simulink model "ACC_Scenario_006_cs"  (R2014b)
settings: Solver=ode5  SolverMode=SingleTasking  StartTime=0.0  StopTime=inf  FixedStep=1/100  RelTol=1e-3
PreLoadFcn:
  | mbxruntime.callbacks.PreLoadFcn(bdroot);
  | check_NUTS_defined;
  | 
  | assignin('base',['model_closed_' bdroot],false);addpath('../includes_ACC');
PostLoadFcn:
  | mbxruntime.callbacks.PostLoadFcn(bdroot);
InitFcn:
  | mbxruntime.callbacks.InitFcn(bdroot);
StartFcn:
  | mbxruntime.callbacks.StartFcn(bdroot);
StopFcn:
  | mbxruntime.callbacks.StopFcn(bdroot);
model workspace: external: MAT-File .\ACC_Scenario_006_cs_hws.mat (data not in the file)
undefined symbols (not defined in the file or in its folder): mbxruntime, OrientationPitch, OrientationRoll, PositionX, PositionY, PositionZ, tabledata, warningInitialVelocity, x0
undefined symbols (not defined in the file): ACC_Scenario_006_cs_061450488d6753c4, ACC_Scenario_006_cs_13896134c615b72a, ACC_Scenario_006_cs_18eaf2a52f2ef75d, ACC_Scenario_006_cs_59e375456829d2f0, ACC_Scenario_006_cs_8a2109b915871f11, ACC_Scenario_006_cs_a4f79cab717c06e2, ACC_Scenario_006_cs_Audi_A8_1_Dynamics_Simple_initialPitch, ACC_Scenario_006_cs_Audi_A8_1_Dynamics_Simple_initialRoll, ACC_Scenario_006_cs_Audi_A8_1_Dynamics_Simple_initialX, ACC_Scenario_006_cs_Audi_A8_1_Dynamics_Simple_initialY, ACC_Scenario_006_cs_Audi_A8_1_Dynamics_Simple_initialYaw, ACC_Scenario_006_cs_Audi_A8_1_Dynamics_Simple_initialZ, ACC_Scenario_006_cs_BMW_X5_1_Path_pathUniqueID, ACC_Scenario_006_cs_BMW_X5_1_SpeedProfile_speedProfileUniqueID, ACC_Scenario_006_cs_e4633c18fd34a832, ACC_Scenario_006_cs_f83c81dc10cd364a, ACC_Scenario_006_cs_Fiat_Bravo_1_Path_pathUniqueID, ACC_Scenario_006_cs_Ford_Fiesta_1_Path_pathUniqueID, ACC_Scenario_006_cs_Honda_Pan_European_1_Path_pathUniqueID, ACC_Scenario_006_cs_Mazda_RX8_1_Path_pathUniqueID, ACC_Scenario_006_cs_Sphere_1_Dynamics_Empty_STATE_Sphere_1_x0, ACC_Scenario_006_cs_Sphere_1_Dynamics_Empty_STATE_Sphere_1_y0, ACC_Scenario_006_cs_Sphere_1_Dynamics_Empty_STATE_Sphere_1_Yaw0, ACC_Scenario_006_cs_Sphere_1_Dynamics_Empty_STATE_Sphere_1_z0, ACC_Scenario_006_cs_Toyota_Yaris_1_Path_pathUniqueID, SteeringColumn, SteeringWheel, Wheel0, Wheel0_Suspension, Wheel1, Wheel1_Suspension, WheelL0, WheelL1, WheelR0, WheelR1
libraries: simulink_extras x60, simulink x21, PreScanSimulinkLibrary x5, PreScanUsefulBlocks x2
(part 16 of 24)

== system ACC_Scenario_006_cs/VISUMatrixSign_HighwayOverhang_1/Actuator ==
  VISUMatrixSign_HighwayOverhang_1 : Inport  Tag=inport/VisuMatrixSign  SampleTime=1/100  BusOutputAsStruct=on
  DemuxVisuMatrixSign : Demux  Outputs=2
  visu_MatrixSign_1 : S-Function  FunctionName=sfun_ResourceNameSelector  Parameters=mbxruntime.parameters.convert(UniqueID), mbxruntime.parameters.convert(ResourceList), mbxruntime.parameters.convert(PivotName),tabledata, TimeStep  EnableBusSupport=off  mask(PreScan Sink Block: VisuMatrixSign){UniqueID=109, ResourceList={'1' 'InformationSign\MatrixSign_GreenArrow.png' '2' 'InformationSign\sign1.jpg' '3' 'InformationSign\sign2.jpg' '4' 'InformationSign\sign3.jpg' '5' 'InformationSign\sign10.png' '7' 'InformationSign\SEARCH_Logo.png' '8' 'InformationSign\sharp_edges.jpg' '9' 'InformationSign\road_surprises.jpg' '10' 'InformationSign\sign5.JPG' '11' 'InformationSign\tacos.jpg' '12' 'InformationSign\dont_even_think.jpg' '13' 'InformationSign\cthulhuwarn.jpg' '14' 'InformationSign\sign7.JPG' '15' 'InformationSign\sign32.jpg' '16' 'InformationSign\NoParking.jpg' '17' 'InformationSign\TheFuture.jpg' '18' 'InformationSign\sign4.jpg' '19' 'InformationSign\sign31.jpg' '20' 'InformationSign\Empty.jpeg' }, PivotName=/child:name=MatrixSign_1/trafficSignElement, TimeStep=1/100}
      mask prompts: UniqueID "Parent Unique Identifier (auto-generated)"; ResourceList "Resource List (auto-generated)"; PivotName "Name of pivot (auto-generated)"; TimeStep "Simulink time step"
      mask help:
      | The VisuMatrixSign block provides a way to adapt the texture of the plates connected to an overhang, based on Resource IDs of the texture files.
      |
      | For more information, please click Help.
      mask init:
      | [tabledata] = mbxruntime.parameters.table(UniqueID,ResourceList,PivotName);
      mask Help: eval('openHelp(733)')
      mask Display: image(imread('HighwaySpeedMatrix.png'))
  visu_MatrixSign_2 : S-Function  FunctionName=sfun_ResourceNameSelector  Parameters=mbxruntime.parameters.convert(UniqueID), mbxruntime.parameters.convert(ResourceList), mbxruntime.parameters.convert(PivotName),tabledata, TimeStep  EnableBusSupport=off  mask(PreScan Sink Block: VisuMatrixSign){UniqueID=109, ResourceList={'1' 'InformationSign\MatrixSign_GreenArrow.png' '2' 'InformationSign\sign1.jpg' '3' 'InformationSign\sign2.jpg' '4' 'InformationSign\sign3.jpg' '5' 'InformationSign\sign10.png' '7' 'InformationSign\SEARCH_Logo.png' '8' 'InformationSign\sharp_edges.jpg' '9' 'InformationSign\road_surprises.jpg' '10' 'InformationSign\sign5.JPG' '11' 'InformationSign\tacos.jpg' '12' 'InformationSign\dont_even_think.jpg' '13' 'InformationSign\cthulhuwarn.jpg' '14' 'InformationSign\sign7.JPG' '15' 'InformationSign\sign32.jpg' '16' 'InformationSign\NoParking.jpg' '17' 'InformationSign\TheFuture.jpg' '18' 'InformationSign\sign4.jpg' '19' 'InformationSign\sign31.jpg' '20' 'InformationSign\Empty.jpeg' }, PivotName=/child:name=MatrixSign_2/trafficSignElement, TimeStep=1/100}
      mask prompts: UniqueID "Parent Unique Identifier (auto-generated)"; ResourceList "Resource List (auto-generated)"; PivotName "Name of pivot (auto-generated)"; TimeStep "Simulink time step"
      mask help:
      | The VisuMatrixSign block provides a way to adapt the texture of the plates connected to an overhang, based on Resource IDs of the texture files.
      |
      | For more information, please click Help.
      mask init:
      | [tabledata] = mbxruntime.parameters.table(UniqueID,ResourceList,PivotName);
      mask Help: eval('openHelp(733)')
      mask Display: image(imread('HighwaySpeedMatrix.png'))
  wires:
  VISUMatrixSign_HighwayOverhang_1/1 -> DemuxVisuMatrixSign/1
  DemuxVisuMatrixSign/1 -> visu_MatrixSign_1/1
  DemuxVisuMatrixSign/2 -> visu_MatrixSign_2/1

== system ACC_Scenario_006_cs/VISUMatrixSign_HighwayOverhang_10/Actuator ==
  VISUMatrixSign_HighwayOverhang_10 : Inport  Tag=inport/VisuMatrixSign  SampleTime=1/100  BusOutputAsStruct=on
  DemuxVisuMatrixSign : Demux  Outputs=2
  visu_InformationPlate_15 : S-Function  FunctionName=sfun_ResourceNameSelector  Parameters=mbxruntime.parameters.convert(UniqueID), mbxruntime.parameters.convert(ResourceList), mbxruntime.parameters.convert(PivotName),tabledata, TimeStep  EnableBusSupport=off  mask(PreScan Sink Block: VisuMatrixSign){UniqueID=119, ResourceList={'1' 'InformationSign\MatrixSign_GreenArrow.png' '2' 'InformationSign\sign1.jpg' '3' 'InformationSign\sign2.jpg' '4' 'InformationSign\sign3.jpg' '5' 'InformationSign\sign10.png' '7' 'InformationSign\SEARCH_Logo.png' '8' 'InformationSign\sharp_edges.jpg' '9' 'InformationSign\road_surprises.jpg' '10' 'InformationSign\sign5.JPG' '11' 'InformationSign\tacos.jpg' '12' 'InformationSign\dont_even_think.jpg' '13' 'InformationSign\cthulhuwarn.jpg' '14' 'InformationSign\sign7.JPG' '15' 'InformationSign\sign32.jpg' '16' 'InformationSign\NoParking.jpg' '17' 'InformationSign\TheFuture.jpg' '18' 'InformationSign\sign4.jpg' '19' 'InformationSign\sign31.jpg' '20' 'InformationSign\Empty.jpeg' }, PivotName=/child:name=HighwayOverhang_10.InformationPlate_15/trafficSignElement, TimeStep=1/100}
      mask prompts: UniqueID "Parent Unique Identifier (auto-generated)"; ResourceList "Resource List (auto-generated)"; PivotName "Name of pivot (auto-generated)"; TimeStep "Simulink time step"
      mask help:
      | The VisuMatrixSign block provides a way to adapt the texture of the plates connected to an overhang, based on Resource IDs of the texture files.
      |
      | For more information, please click Help.
      mask init:
      | [tabledata] = mbxruntime.parameters.table(UniqueID,ResourceList,PivotName);
      mask Help: eval('openHelp(733)')
      mask Display: image(imread('HighwaySpeedMatrix.png'))
  visu_InformationPlate_16 : S-Function  FunctionName=sfun_ResourceNameSelector  Parameters=mbxruntime.parameters.convert(UniqueID), mbxruntime.parameters.convert(ResourceList), mbxruntime.parameters.convert(PivotName),tabledata, TimeStep  EnableBusSupport=off  mask(PreScan Sink Block: VisuMatrixSign){UniqueID=119, ResourceList={'1' 'InformationSign\MatrixSign_GreenArrow.png' '2' 'InformationSign\sign1.jpg' '3' 'InformationSign\sign2.jpg' '4' 'InformationSign\sign3.jpg' '5' 'InformationSign\sign10.png' '7' 'InformationSign\SEARCH_Logo.png' '8' 'InformationSign\sharp_edges.jpg' '9' 'InformationSign\road_surprises.jpg' '10' 'InformationSign\sign5.JPG' '11' 'InformationSign\tacos.jpg' '12' 'InformationSign\dont_even_think.jpg' '13' 'InformationSign\cthulhuwarn.jpg' '14' 'InformationSign\sign7.JPG' '15' 'InformationSign\sign32.jpg' '16' 'InformationSign\NoParking.jpg' '17' 'InformationSign\TheFuture.jpg' '18' 'InformationSign\sign4.jpg' '19' 'InformationSign\sign31.jpg' '20' 'InformationSign\Empty.jpeg' }, PivotName=/child:name=HighwayOverhang_10.InformationPlate_16/trafficSignElement, TimeStep=1/100}
      mask prompts: UniqueID "Parent Unique Identifier (auto-generated)"; ResourceList "Resource List (auto-generated)"; PivotName "Name of pivot (auto-generated)"; TimeStep "Simulink time step"
      mask help:
      | The VisuMatrixSign block provides a way to adapt the texture of the plates connected to an overhang, based on Resource IDs of the texture files.
      |
      | For more information, please click Help.
      mask init:
      | [tabledata] = mbxruntime.parameters.table(UniqueID,ResourceList,PivotName);
      mask Help: eval('openHelp(733)')
      mask Display: image(imread('HighwaySpeedMatrix.png'))
  wires:
  VISUMatrixSign_HighwayOverhang_10/1 -> DemuxVisuMatrixSign/1
  DemuxVisuMatrixSign/1 -> visu_InformationPlate_15/1
  DemuxVisuMatrixSign/2 -> visu_InformationPlate_16/1

== system ACC_Scenario_006_cs/VISUMatrixSign_HighwayOverhang_11/Actuator ==
  VISUMatrixSign_HighwayOverhang_11 : Inport  Tag=inport/VisuMatrixSign  SampleTime=1/100  BusOutputAsStruct=on
  DemuxVisuMatrixSign : Demux  Outputs=2
  visu_MatrixSign_7 : S-Function  FunctionName=sfun_ResourceNameSelector  Parameters=mbxruntime.parameters.convert(UniqueID), mbxruntime.parameters.convert(ResourceList), mbxruntime.parameters.convert(PivotName),tabledata, TimeStep  EnableBusSupport=off  mask(PreScan Sink Block: VisuMatrixSign){UniqueID=120, ResourceList={'1' 'InformationSign\MatrixSign_GreenArrow.png' '2' 'InformationSign\sign1.jpg' '3' 'InformationSign\sign2.jpg' '4' 'InformationSign\sign3.jpg' '5' 'InformationSign\sign10.png' '7' 'InformationSign\SEARCH_Logo.png' '8' 'InformationSign\sharp_edges.jpg' '9' 'InformationSign\road_surprises.jpg' '10' 'InformationSign\sign5.JPG' '11' 'InformationSign\tacos.jpg' '12' 'InformationSign\dont_even_think.jpg' '13' 'InformationSign\cthulhuwarn.jpg' '14' 'InformationSign\sign7.JPG' '15' 'InformationSign\sign32.jpg' '16' 'InformationSign\NoParking.jpg' '17' 'InformationSign\TheFuture.jpg' '18' 'InformationSign\sign4.jpg' '19' 'InformationSign\sign31.jpg' '20' 'InformationSign\Empty.jpeg' }, PivotName=/child:name=MatrixSign_7/trafficSignElement, TimeStep=1/100}
      mask prompts: UniqueID "Parent Unique Identifier (auto-generated)"; ResourceList "Resource List (auto-generated)"; PivotName "Name of pivot (auto-generated)"; TimeStep "Simulink time step"
      mask help:
      | The VisuMatrixSign block provides a way to adapt the texture of the plates connected to an overhang, based on Resource IDs of the texture files.
      |
      | For more information, please click Help.
      mask init:
      | [tabledata] = mbxruntime.parameters.table(UniqueID,ResourceList,PivotName);
      mask Help: eval('openHelp(733)')
      mask Display: image(imread('HighwaySpeedMatrix.png'))
  visu_MatrixSign_8 : S-Function  FunctionName=sfun_ResourceNameSelector  Parameters=mbxruntime.parameters.convert(UniqueID), mbxruntime.parameters.convert(ResourceList), mbxruntime.parameters.convert(PivotName),tabledata, TimeStep  EnableBusSupport=off  mask(PreScan Sink Block: VisuMatrixSign){UniqueID=120, ResourceList={'1' 'InformationSign\MatrixSign_GreenArrow.png' '2' 'InformationSign\sign1.jpg' '3' 'InformationSign\sign2.jpg' '4' 'InformationSign\sign3.jpg' '5' 'InformationSign\sign10.png' '7' 'InformationSign\SEARCH_Logo.png' '8' 'InformationSign\sharp_edges.jpg' '9' 'InformationSign\road_surprises.jpg' '10' 'InformationSign\sign5.JPG' '11' 'InformationSign\tacos.jpg' '12' 'InformationSign\dont_even_think.jpg' '13' 'InformationSign\cthulhuwarn.jpg' '14' 'InformationSign\sign7.JPG' '15' 'InformationSign\sign32.jpg' '16' 'InformationSign\NoParking.jpg' '17' 'InformationSign\TheFuture.jpg' '18' 'InformationSign\sign4.jpg' '19' 'InformationSign\sign31.jpg' '20' 'InformationSign\Empty.jpeg' }, PivotName=/child:name=MatrixSign_8/trafficSignElement, TimeStep=1/100}
      mask prompts: UniqueID "Parent Unique Identifier (auto-generated)"; ResourceList "Resource List (auto-generated)"; PivotName "Name of pivot (auto-generated)"; TimeStep "Simulink time step"
      mask help:
      | The VisuMatrixSign block provides a way to adapt the texture of the plates connected to an overhang, based on Resource IDs of the texture files.
      |
      | For more information, please click Help.
      mask init:
      | [tabledata] = mbxruntime.parameters.table(UniqueID,ResourceList,PivotName);
      mask Help: eval('openHelp(733)')
      mask Display: image(imread('HighwaySpeedMatrix.png'))
  wires:
  VISUMatrixSign_HighwayOverhang_11/1 -> DemuxVisuMatrixSign/1
  DemuxVisuMatrixSign/1 -> visu_MatrixSign_7/1
  DemuxVisuMatrixSign/2 -> visu_MatrixSign_8/1

== system ACC_Scenario_006_cs/VISUMatrixSign_HighwayOverhang_12/Actuator ==
  VISUMatrixSign_HighwayOverhang_12 : Inport  Tag=inport/VisuMatrixSign  SampleTime=1/100  BusOutputAsStruct=on
  DemuxVisuMatrixSign : Demux  Outputs=2
  visu_MatrixSign_5 : S-Function  FunctionName=sfun_ResourceNameSelector  Parameters=mbxruntime.parameters.convert(UniqueID), mbxruntime.parameters.convert(ResourceList), mbxruntime.parameters.convert(PivotName),tabledata, TimeStep  EnableBusSupport=off  mask(PreScan Sink Block: VisuMatrixSign){UniqueID=121, ResourceList={'1' 'InformationSign\MatrixSign_GreenArrow.png' '2' 'InformationSign\sign1.jpg' '3' 'InformationSign\sign2.jpg' '4' 'InformationSign\sign3.jpg' '5' 'InformationSign\sign10.png' '7' 'InformationSign\SEARCH_Logo.png' '8' 'InformationSign\sharp_edges.jpg' '9' 'InformationSign\road_surprises.jpg' '10' 'InformationSign\sign5.JPG' '11' 'InformationSign\tacos.jpg' '12' 'InformationSign\dont_even_think.jpg' '13' 'InformationSign\cthulhuwarn.jpg' '14' 'InformationSign\sign7.JPG' '15' 'InformationSign\sign32.jpg' '16' 'InformationSign\NoParking.jpg' '17' 'InformationSign\TheFuture.jpg' '18' 'InformationSign\sign4.jpg' '19' 'InformationSign\sign31.jpg' '20' 'InformationSign\Empty.jpeg' }, PivotName=/child:name=MatrixSign_5/trafficSignElement, TimeStep=1/100}
      mask prompts: UniqueID "Parent Unique Identifier (auto-generated)"; ResourceList "Resource List (auto-generated)"; PivotName "Name of pivot (auto-generated)"; TimeStep "Simulink time step"
      mask help:
      | The VisuMatrixSign block provides a way to adapt the texture of the plates connected to an overhang, based on Resource IDs of the texture files.
      |
      | For more information, please click Help.
      mask init:
      | [tabledata] = mbxruntime.parameters.table(UniqueID,ResourceList,PivotName);
      mask Help: eval('openHelp(733)')
      mask Display: image(imread('HighwaySpeedMatrix.png'))
  visu_MatrixSign_6 : S-Function  FunctionName=sfun_ResourceNameSelector  Parameters=mbxruntime.parameters.convert(UniqueID), mbxruntime.parameters.convert(ResourceList), mbxruntime.parameters.convert(PivotName),tabledata, TimeStep  EnableBusSupport=off  mask(PreScan Sink Block: VisuMatrixSign){UniqueID=121, ResourceList={'1' 'InformationSign\MatrixSign_GreenArrow.png' '2' 'InformationSign\sign1.jpg' '3' 'InformationSign\sign2.jpg' '4' 'InformationSign\sign3.jpg' '5' 'InformationSign\sign10.png' '7' 'InformationSign\SEARCH_Logo.png' '8' 'InformationSign\sharp_edges.jpg' '9' 'InformationSign\road_surprises.jpg' '10' 'InformationSign\sign5.JPG' '11' 'InformationSign\tacos.jpg' '12' 'InformationSign\dont_even_think.jpg' '13' 'InformationSign\cthulhuwarn.jpg' '14' 'InformationSign\sign7.JPG' '15' 'InformationSign\sign32.jpg' '16' 'InformationSign\NoParking.jpg' '17' 'InformationSign\TheFuture.jpg' '18' 'InformationSign\sign4.jpg' '19' 'InformationSign\sign31.jpg' '20' 'InformationSign\Empty.jpeg' }, PivotName=/child:name=MatrixSign_6/trafficSignElement, TimeStep=1/100}
      mask prompts: UniqueID "Parent Unique Identifier (auto-generated)"; ResourceList "Resource List (auto-generated)"; PivotName "Name of pivot (auto-generated)"; TimeStep "Simulink time step"
      mask help:
      | The VisuMatrixSign block provides a way to adapt the texture of the plates connected to an overhang, based on Resource IDs of the texture files.
      |
      | For more information, please click Help.
      mask init:
      | [tabledata] = mbxruntime.parameters.table(UniqueID,ResourceList,PivotName);
      mask Help: eval('openHelp(733)')
      mask Display: image(imread('HighwaySpeedMatrix.png'))
  wires:
  VISUMatrixSign_HighwayOverhang_12/1 -> DemuxVisuMatrixSign/1
  DemuxVisuMatrixSign/1 -> visu_MatrixSign_5/1
  DemuxVisuMatrixSign/2 -> visu_MatrixSign_6/1

== system ACC_Scenario_006_cs/VISUMatrixSign_HighwayOverhang_2/Actuator ==
  VISUMatrixSign_HighwayOverhang_2 : Inport  Tag=inport/VisuMatrixSign  SampleTime=1/100  BusOutputAsStruct=on
  DemuxVisuMatrixSign : Demux  Outputs=2
  visu_MatrixSign_3 : S-Function  FunctionName=sfun_ResourceNameSelector  Parameters=mbxruntime.parameters.convert(UniqueID), mbxruntime.parameters.convert(ResourceList), mbxruntime.parameters.convert(PivotName),tabledata, TimeStep  EnableBusSupport=off  mask(PreScan Sink Block: VisuMatrixSign){UniqueID=110, ResourceList={'1' 'InformationSign\MatrixSign_GreenArrow.png' '2' 'InformationSign\sign1.jpg' '3' 'InformationSign\sign2.jpg' '4' 'InformationSign\sign3.jpg' '5' 'InformationSign\sign10.png' '7' 'InformationSign\SEARCH_Logo.png' '8' 'InformationSign\sharp_edges.jpg' '9' 'InformationSign\road_surprises.jpg' '10' 'InformationSign\sign5.JPG' '11' 'InformationSign\tacos.jpg' '12' 'InformationSign\dont_even_think.jpg' '13' 'InformationSign\cthulhuwarn.jpg' '14' 'InformationSign\sign7.JPG' '15' 'InformationSign\sign32.jpg' '16' 'InformationSign\NoParking.jpg' '17' 'InformationSign\TheFuture.jpg' '18' 'InformationSign\sign4.jpg' '19' 'InformationSign\sign31.jpg' '20' 'InformationSign\Empty.jpeg' }, PivotName=/child:name=MatrixSign_3/trafficSignElement, TimeStep=1/100}
      mask prompts: UniqueID "Parent Unique Identifier (auto-generated)"; ResourceList "Resource List (auto-generated)"; PivotName "Name of pivot (auto-generated)"; TimeStep "Simulink time step"
      mask help:
      | The VisuMatrixSign block provides a way to adapt the texture of the plates connected to an overhang, based on Resource IDs of the texture files.
      |
      | For more information, please click Help.
      mask init:
      | [tabledata] = mbxruntime.parameters.table(UniqueID,ResourceList,PivotName);
      mask Help: eval('openHelp(733)')
      mask Display: image(imread('HighwaySpeedMatrix.png'))
  visu_MatrixSign_4 : S-Function  FunctionName=sfun_ResourceNameSelector  Parameters=mbxruntime.parameters.convert(UniqueID), mbxruntime.parameters.convert(ResourceList), mbxruntime.parameters.convert(PivotName),tabledata, TimeStep  EnableBusSupport=off  mask(PreScan Sink Block: VisuMatrixSign){UniqueID=110, ResourceList={'1' 'InformationSign\MatrixSign_GreenArrow.png' '2' 'InformationSign\sign1.jpg' '3' 'InformationSign\sign2.jpg' '4' 'InformationSign\sign3.jpg' '5' 'InformationSign\sign10.png' '7' 'InformationSign\SEARCH_Logo.png' '8' 'InformationSign\sharp_edges.jpg' '9' 'InformationSign\road_surprises.jpg' '10' 'InformationSign\sign5.JPG' '11' 'InformationSign\tacos.jpg' '12' 'InformationSign\dont_even_think.jpg' '13' 'InformationSign\cthulhuwarn.jpg' '14' 'InformationSign\sign7.JPG' '15' 'InformationSign\sign32.jpg' '16' 'InformationSign\NoParking.jpg' '17' 'InformationSign\TheFuture.jpg' '18' 'InformationSign\sign4.jpg' '19' 'InformationSign\sign31.jpg' '20' 'InformationSign\Empty.jpeg' }, PivotName=/child:name=MatrixSign_4/trafficSignElement, TimeStep=1/100}
      mask prompts: UniqueID "Parent Unique Identifier (auto-generated)"; ResourceList "Resource List (auto-generated)"; PivotName "Name of pivot (auto-generated)"; TimeStep "Simulink time step"
      mask help:
      | The VisuMatrixSign block provides a way to adapt the texture of the plates connected to an overhang, based on Resource IDs of the texture files.
      |
      | For more information, please click Help.
      mask init:
      | [tabledata] = mbxruntime.parameters.table(UniqueID,ResourceList,PivotName);
      mask Help: eval('openHelp(733)')
      mask Display: image(imread('HighwaySpeedMatrix.png'))
  wires:
  VISUMatrixSign_HighwayOverhang_2/1 -> DemuxVisuMatrixSign/1
  DemuxVisuMatrixSign/1 -> visu_MatrixSign_3/1
  DemuxVisuMatrixSign/2 -> visu_MatrixSign_4/1

== system ACC_Scenario_006_cs/VISUMatrixSign_HighwayOverhang_3/Actuator ==
  VISUMatrixSign_HighwayOverhang_3 : Inport  Tag=inport/VisuMatrixSign  SampleTime=1/100  BusOutputAsStruct=on
  DemuxVisuMatrixSign : Demux  Outputs=2
  visu_InformationPlate_1 : S-Function  FunctionName=sfun_ResourceNameSelector  Parameters=mbxruntime.parameters.convert(UniqueID), mbxruntime.parameters.convert(ResourceList), mbxruntime.parameters.convert(PivotName),tabledata, TimeStep  EnableBusSupport=off  mask(PreScan Sink Block: VisuMatrixSign){UniqueID=112, ResourceList={'1' 'InformationSign\MatrixSign_GreenArrow.png' '2' 'InformationSign\sign1.jpg' '3' 'InformationSign\sign2.jpg' '4' 'InformationSign\sign3.jpg' '5' 'InformationSign\sign10.png' '7' 'InformationSign\SEARCH_Logo.png' '8' 'InformationSign\sharp_edges.jpg' '9' 'InformationSign\road_surprises.jpg' '10' 'InformationSign\sign5.JPG' '11' 'InformationSign\tacos.jpg' '12' 'InformationSign\dont_even_think.jpg' '13' 'InformationSign\cthulhuwarn.jpg' '14' 'InformationSign\sign7.JPG' '15' 'InformationSign\sign32.jpg' '16' 'InformationSign\NoParking.jpg' '17' 'InformationSign\TheFuture.jpg' '18' 'InformationSign\sign4.jpg' '19' 'InformationSign\sign31.jpg' '20' 'InformationSign\Empty.jpeg' }, PivotName=/child:name=HighwayOverhang_3.InformationPlate_1/trafficSignElement, TimeStep=1/100}
      mask prompts: UniqueID "Parent Unique Identifier (auto-generated)"; ResourceList "Resource List (auto-generated)"; PivotName "Name of pivot (auto-generated)"; TimeStep "Simulink time step"
      mask help:
      | The VisuMatrixSign block provides a way to adapt the texture of the plates connected to an overhang, based on Resource IDs of the texture files.
      |
      | For more information, please click Help.
      mask init:
      | [tabledata] = mbxruntime.parameters.table(UniqueID,ResourceList,PivotName);
      mask Help: eval('openHelp(733)')
      mask Display: image(imread('HighwaySpeedMatrix.png'))
  visu_InformationPlate_2 : S-Function  FunctionName=sfun_ResourceNameSelector  Parameters=mbxruntime.parameters.convert(UniqueID), mbxruntime.parameters.convert(ResourceList), mbxruntime.parameters.convert(PivotName),tabledata, TimeStep  EnableBusSupport=off  mask(PreScan Sink Block: VisuMatrixSign){UniqueID=112, ResourceList={'1' 'InformationSign\MatrixSign_GreenArrow.png' '2' 'InformationSign\sign1.jpg' '3' 'InformationSign\sign2.jpg' '4' 'InformationSign\sign3.jpg' '5' 'InformationSign\sign10.png' '7' 'InformationSign\SEARCH_Logo.png' '8' 'InformationSign\sharp_edges.jpg' '9' 'InformationSign\road_surprises.jpg' '10' 'InformationSign\sign5.JPG' '11' 'InformationSign\tacos.jpg' '12' 'InformationSign\dont_even_think.jpg' '13' 'InformationSign\cthulhuwarn.jpg' '14' 'InformationSign\sign7.JPG' '15' 'InformationSign\sign32.jpg' '16' 'InformationSign\NoParking.jpg' '17' 'InformationSign\TheFuture.jpg' '18' 'InformationSign\sign4.jpg' '19' 'InformationSign\sign31.jpg' '20' 'InformationSign\Empty.jpeg' }, PivotName=/child:name=HighwayOverhang_3.InformationPlate_2/trafficSignElement, TimeStep=1/100}
      mask prompts: UniqueID "Parent Unique Identifier (auto-generated)"; ResourceList "Resource List (auto-generated)"; PivotName "Name of pivot (auto-generated)"; TimeStep "Simulink time step"
      mask help:
      | The VisuMatrixSign block provides a way to adapt the texture of the plates connected to an overhang, based on Resource IDs of the texture files.
      |
      | For more information, please click Help.
      mask init:
      | [tabledata] = mbxruntime.parameters.table(UniqueID,ResourceList,PivotName);
      mask Help: eval('openHelp(733)')
      mask Display: image(imread('HighwaySpeedMatrix.png'))
  wires:
  VISUMatrixSign_HighwayOverhang_3/1 -> DemuxVisuMatrixSign/1
  DemuxVisuMatrixSign/1 -> visu_InformationPlate_1/1
  DemuxVisuMatrixSign/2 -> visu_InformationPlate_2/1

== system ACC_Scenario_006_cs/VISUMatrixSign_HighwayOverhang_4/Actuator ==
  VISUMatrixSign_HighwayOverhang_4 : Inport  Tag=inport/VisuMatrixSign  SampleTime=1/100  BusOutputAsStruct=on
  DemuxVisuMatrixSign : Demux  Outputs=2
  visu_InformationPlate_3 : S-Function  FunctionName=sfun_ResourceNameSelector  Parameters=mbxruntime.parameters.convert(UniqueID), mbxruntime.parameters.convert(ResourceList), mbxruntime.parameters.convert(PivotName),tabledata, TimeStep  EnableBusSupport=off  mask(PreScan Sink Block: VisuMatrixSign){UniqueID=113, ResourceList={'1' 'InformationSign\MatrixSign_GreenArrow.png' '2' 'InformationSign\sign1.jpg' '3' 'InformationSign\sign2.jpg' '4' 'InformationSign\sign3.jpg' '5' 'InformationSign\sign10.png' '7' 'InformationSign\SEARCH_Logo.png' '8' 'InformationSign\sharp_edges.jpg' '9' 'InformationSign\road_surprises.jpg' '10' 'InformationSign\sign5.JPG' '11' 'InformationSign\tacos.jpg' '12' 'InformationSign\dont_even_think.jpg' '13' 'InformationSign\cthulhuwarn.jpg' '14' 'InformationSign\sign7.JPG' '15' 'InformationSign\sign32.jpg' '16' 'InformationSign\NoParking.jpg' '17' 'InformationSign\TheFuture.jpg' '18' 'InformationSign\sign4.jpg' '19' 'InformationSign\sign31.jpg' '20' 'InformationSign\Empty.jpeg' }, PivotName=/child:name=HighwayOverhang_4.InformationPlate_3/trafficSignElement, TimeStep=1/100}
      mask prompts: UniqueID "Parent Unique Identifier (auto-generated)"; ResourceList "Resource List (auto-generated)"; PivotName "Name of pivot (auto-generated)"; TimeStep "Simulink time step"
      mask help:
      | The VisuMatrixSign block provides a way to adapt the texture of the plates connected to an overhang, based on Resource IDs of the texture files.
      |
      | For more information, please click Help.
      mask init:
      | [tabledata] = mbxruntime.parameters.table(UniqueID,ResourceList,PivotName);
      mask Help: eval('openHelp(733)')
      mask Display: image(imread('HighwaySpeedMatrix.png'))
  visu_InformationPlate_4 : S-Function  FunctionName=sfun_ResourceNameSelector  Parameters=mbxruntime.parameters.convert(UniqueID), mbxruntime.parameters.convert(ResourceList), mbxruntime.parameters.convert(PivotName),tabledata, TimeStep  EnableBusSupport=off  mask(PreScan Sink Block: VisuMatrixSign){UniqueID=113, ResourceList={'1' 'InformationSign\MatrixSign_GreenArrow.png' '2' 'InformationSign\sign1.jpg' '3' 'InformationSign\sign2.jpg' '4' 'InformationSign\sign3.jpg' '5' 'InformationSign\sign10.png' '7' 'InformationSign\SEARCH_Logo.png' '8' 'InformationSign\sharp_edges.jpg' '9' 'InformationSign\road_surprises.jpg' '10' 'InformationSign\sign5.JPG' '11' 'InformationSign\tacos.jpg' '12' 'InformationSign\dont_even_think.jpg' '13' 'InformationSign\cthulhuwarn.jpg' '14' 'InformationSign\sign7.JPG' '15' 'InformationSign\sign32.jpg' '16' 'InformationSign\NoParking.jpg' '17' 'InformationSign\TheFuture.jpg' '18' 'InformationSign\sign4.jpg' '19' 'InformationSign\sign31.jpg' '20' 'InformationSign\Empty.jpeg' }, PivotName=/child:name=HighwayOverhang_4.InformationPlate_4/trafficSignElement, TimeStep=1/100}
      mask prompts: UniqueID "Parent Unique Identifier (auto-generated)"; ResourceList "Resource List (auto-generated)"; PivotName "Name of pivot (auto-generated)"; TimeStep "Simulink time step"
      mask help:
      | The VisuMatrixSign block provides a way to adapt the texture of the plates connected to an overhang, based on Resource IDs of the texture files.
      |
      | For more information, please click Help.
      mask init:
      | [tabledata] = mbxruntime.parameters.table(UniqueID,ResourceList,PivotName);
      mask Help: eval('openHelp(733)')
      mask Display: image(imread('HighwaySpeedMatrix.png'))
  wires:
  VISUMatrixSign_HighwayOverhang_4/1 -> DemuxVisuMatrixSign/1
  DemuxVisuMatrixSign/1 -> visu_InformationPlate_3/1
  DemuxVisuMatrixSign/2 -> visu_InformationPlate_4/1

== system ACC_Scenario_006_cs/VISUMatrixSign_HighwayOverhang_5/Actuator ==
  VISUMatrixSign_HighwayOverhang_5 : Inport  Tag=inport/VisuMatrixSign  SampleTime=1/100  BusOutputAsStruct=on
  DemuxVisuMatrixSign : Demux  Outputs=2
  visu_InformationPlate_5 : S-Function  FunctionName=sfun_ResourceNameSelector  Parameters=mbxruntime.parameters.convert(UniqueID), mbxruntime.parameters.convert(ResourceList), mbxruntime.parameters.convert(PivotName),tabledata, TimeStep  EnableBusSupport=off  mask(PreScan Sink Block: VisuMatrixSign){UniqueID=114, ResourceList={'1' 'InformationSign\MatrixSign_GreenArrow.png' '2' 'InformationSign\sign1.jpg' '3' 'InformationSign\sign2.jpg' '4' 'InformationSign\sign3.jpg' '5' 'InformationSign\sign10.png' '7' 'InformationSign\SEARCH_Logo.png' '8' 'InformationSign\sharp_edges.jpg' '9' 'InformationSign\road_surprises.jpg' '10' 'InformationSign\sign5.JPG' '11' 'InformationSign\tacos.jpg' '12' 'InformationSign\dont_even_think.jpg' '13' 'InformationSign\cthulhuwarn.jpg' '14' 'InformationSign\sign7.JPG' '15' 'InformationSign\sign32.jpg' '16' 'InformationSign\NoParking.jpg' '17' 'InformationSign\TheFuture.jpg' '18' 'InformationSign\sign4.jpg' '19' 'InformationSign\sign31.jpg' '20' 'InformationSign\Empty.jpeg' }, PivotName=/child:name=HighwayOverhang_5.InformationPlate_5/trafficSignElement, TimeStep=1/100}
      mask prompts: UniqueID "Parent Unique Identifier (auto-generated)"; ResourceList "Resource List (auto-generated)"; PivotName "Name of pivot (auto-generated)"; TimeStep "Simulink time step"
      mask help:
      | The VisuMatrixSign block provides a way to adapt the texture of the plates connected to an overhang, based on Resource IDs of the texture files.
      |
      | For more information, please click Help.
      mask init:
      | [tabledata] = mbxruntime.parameters.table(UniqueID,ResourceList,PivotName);
      mask Help: eval('openHelp(733)')
      mask Display: image(imread('HighwaySpeedMatrix.png'))
  visu_InformationPlate_6 : S-Function  FunctionName=sfun_ResourceNameSelector  Parameters=mbxruntime.parameters.convert(UniqueID), mbxruntime.parameters.convert(ResourceList), mbxruntime.parameters.convert(PivotName),tabledata, TimeStep  EnableBusSupport=off  mask(PreScan Sink Block: VisuMatrixSign){UniqueID=114, ResourceList={'1' 'InformationSign\MatrixSign_GreenArrow.png' '2' 'InformationSign\sign1.jpg' '3' 'InformationSign\sign2.jpg' '4' 'InformationSign\sign3.jpg' '5' 'InformationSign\sign10.png' '7' 'InformationSign\SEARCH_Logo.png' '8' 'InformationSign\sharp_edges.jpg' '9' 'InformationSign\road_surprises.jpg' '10' 'InformationSign\sign5.JPG' '11' 'InformationSign\tacos.jpg' '12' 'InformationSign\dont_even_think.jpg' '13' 'InformationSign\cthulhuwarn.jpg' '14' 'InformationSign\sign7.JPG' '15' 'InformationSign\sign32.jpg' '16' 'InformationSign\NoParking.jpg' '17' 'InformationSign\TheFuture.jpg' '18' 'InformationSign\sign4.jpg' '19' 'InformationSign\sign31.jpg' '20' 'InformationSign\Empty.jpeg' }, PivotName=/child:name=HighwayOverhang_5.InformationPlate_6/trafficSignElement, TimeStep=1/100}
      mask prompts: UniqueID "Parent Unique Identifier (auto-generated)"; ResourceList "Resource List (auto-generated)"; PivotName "Name of pivot (auto-generated)"; TimeStep "Simulink time step"
      mask help:
      | The VisuMatrixSign block provides a way to adapt the texture of the plates connected to an overhang, based on Resource IDs of the texture files.
      |
      | For more information, please click Help.
      mask init:
      | [tabledata] = mbxruntime.parameters.table(UniqueID,ResourceList,PivotName);
      mask Help: eval('openHelp(733)')
      mask Display: image(imread('HighwaySpeedMatrix.png'))
  wires:
  VISUMatrixSign_HighwayOverhang_5/1 -> DemuxVisuMatrixSign/1
  DemuxVisuMatrixSign/1 -> visu_InformationPlate_5/1
  DemuxVisuMatrixSign/2 -> visu_InformationPlate_6/1

== system ACC_Scenario_006_cs/VISUMatrixSign_HighwayOverhang_6/Actuator ==
  VISUMatrixSign_HighwayOverhang_6 : Inport  Tag=inport/VisuMatrixSign  SampleTime=1/100  BusOutputAsStruct=on
  DemuxVisuMatrixSign : Demux  Outputs=2
  visu_InformationPlate_7 : S-Function  FunctionName=sfun_ResourceNameSelector  Parameters=mbxruntime.parameters.convert(UniqueID), mbxruntime.parameters.convert(ResourceList), mbxruntime.parameters.convert(PivotName),tabledata, TimeStep  EnableBusSupport=off  mask(PreScan Sink Block: VisuMatrixSign){UniqueID=115, ResourceList={'1' 'InformationSign\MatrixSign_GreenArrow.png' '2' 'InformationSign\sign1.jpg' '3' 'InformationSign\sign2.jpg' '4' 'InformationSign\sign3.jpg' '5' 'InformationSign\sign10.png' '7' 'InformationSign\SEARCH_Logo.png' '8' 'InformationSign\sharp_edges.jpg' '9' 'InformationSign\road_surprises.jpg' '10' 'InformationSign\sign5.JPG' '11' 'InformationSign\tacos.jpg' '12' 'InformationSign\dont_even_think.jpg' '13' 'InformationSign\cthulhuwarn.jpg' '14' 'InformationSign\sign7.JPG' '15' 'InformationSign\sign32.jpg' '16' 'InformationSign\NoParking.jpg' '17' 'InformationSign\TheFuture.jpg' '18' 'InformationSign\sign4.jpg' '19' 'InformationSign\sign31.jpg' '20' 'InformationSign\Empty.jpeg' }, PivotName=/child:name=HighwayOverhang_6.InformationPlate_7/trafficSignElement, TimeStep=1/100}
      mask prompts: UniqueID "Parent Unique Identifier (auto-generated)"; ResourceList "Resource List (auto-generated)"; PivotName "Name of pivot (auto-generated)"; TimeStep "Simulink time step"
      mask help:
      | The VisuMatrixSign block provides a way to adapt the texture of the plates connected to an overhang, based on Resource IDs of the texture files.
      |
      | For more information, please click Help.
      mask init:
      | [tabledata] = mbxruntime.parameters.table(UniqueID,ResourceList,PivotName);
      mask Help: eval('openHelp(733)')
      mask Display: image(imread('HighwaySpeedMatrix.png'))
  visu_InformationPlate_8 : S-Function  FunctionName=sfun_ResourceNameSelector  Parameters=mbxruntime.parameters.convert(UniqueID), mbxruntime.parameters.convert(ResourceList), mbxruntime.parameters.convert(PivotName),tabledata, TimeStep  EnableBusSupport=off  mask(PreScan Sink Block: VisuMatrixSign){UniqueID=115, ResourceList={'1' 'InformationSign\MatrixSign_GreenArrow.png' '2' 'InformationSign\sign1.jpg' '3' 'InformationSign\sign2.jpg' '4' 'InformationSign\sign3.jpg' '5' 'InformationSign\sign10.png' '7' 'InformationSign\SEARCH_Logo.png' '8' 'InformationSign\sharp_edges.jpg' '9' 'InformationSign\road_surprises.jpg' '10' 'InformationSign\sign5.JPG' '11' 'InformationSign\tacos.jpg' '12' 'InformationSign\dont_even_think.jpg' '13' 'InformationSign\cthulhuwarn.jpg' '14' 'InformationSign\sign7.JPG' '15' 'InformationSign\sign32.jpg' '16' 'InformationSign\NoParking.jpg' '17' 'InformationSign\TheFuture.jpg' '18' 'InformationSign\sign4.jpg' '19' 'InformationSign\sign31.jpg' '20' 'InformationSign\Empty.jpeg' }, PivotName=/child:name=HighwayOverhang_6.InformationPlate_8/trafficSignElement, TimeStep=1/100}
      mask prompts: UniqueID "Parent Unique Identifier (auto-generated)"; ResourceList "Resource List (auto-generated)"; PivotName "Name of pivot (auto-generated)"; TimeStep "Simulink time step"
      mask help:
      | The VisuMatrixSign block provides a way to adapt the texture of the plates connected to an overhang, based on Resource IDs of the texture files.
      |
      | For more information, please click Help.
      mask init:
      | [tabledata] = mbxruntime.parameters.table(UniqueID,ResourceList,PivotName);
      mask Help: eval('openHelp(733)')
      mask Display: image(imread('HighwaySpeedMatrix.png'))
  wires:
  VISUMatrixSign_HighwayOverhang_6/1 -> DemuxVisuMatrixSign/1
  DemuxVisuMatrixSign/1 -> visu_InformationPlate_7/1
  DemuxVisuMatrixSign/2 -> visu_InformationPlate_8/1

== system ACC_Scenario_006_cs/VISUMatrixSign_HighwayOverhang_7/Actuator ==
  VISUMatrixSign_HighwayOverhang_7 : Inport  Tag=inport/VisuMatrixSign  SampleTime=1/100  BusOutputAsStruct=on
  DemuxVisuMatrixSign : Demux  Outputs=2
  visu_InformationPlate_10 : S-Function  FunctionName=sfun_ResourceNameSelector  Parameters=mbxruntime.parameters.convert(UniqueID), mbxruntime.parameters.convert(ResourceList), mbxruntime.parameters.convert(PivotName),tabledata, TimeStep  EnableBusSupport=off  mask(PreScan Sink Block: VisuMatrixSign){UniqueID=116, ResourceList={'1' 'InformationSign\MatrixSign_GreenArrow.png' '2' 'InformationSign\sign1.jpg' '3' 'InformationSign\sign2.jpg' '4' 'InformationSign\sign3.jpg' '5' 'InformationSign\sign10.png' '7' 'InformationSign\SEARCH_Logo.png' '8' 'InformationSign\sharp_edges.jpg' '9' 'InformationSign\road_surprises.jpg' '10' 'InformationSign\sign5.JPG' '11' 'InformationSign\tacos.jpg' '12' 'InformationSign\dont_even_think.jpg' '13' 'InformationSign\cthulhuwarn.jpg' '14' 'InformationSign\sign7.JPG' '15' 'InformationSign\sign32.jpg' '16' 'InformationSign\NoParking.jpg' '17' 'InformationSign\TheFuture.jpg' '18' 'InformationSign\sign4.jpg' '19' 'InformationSign\sign31.jpg' '20' 'InformationSign\Empty.jpeg' }, PivotName=/child:name=HighwayOverhang_7.InformationPlate_10/trafficSignElement, TimeStep=1/100}
      mask prompts: UniqueID "Parent Unique Identifier (auto-generated)"; ResourceList "Resource List (auto-generated)"; PivotName "Name of pivot (auto-generated)"; TimeStep "Simulink time step"
      mask help:
      | The VisuMatrixSign block provides a way to adapt the texture of the plates connected to an overhang, based on Resource IDs of the texture files.
      |
      | For more information, please click Help.
      mask init:
      | [tabledata] = mbxruntime.parameters.table(UniqueID,ResourceList,PivotName);
      mask Help: eval('openHelp(733)')
      mask Display: image(imread('HighwaySpeedMatrix.png'))
  visu_InformationPlate_9 : S-Function  FunctionName=sfun_ResourceNameSelector  Parameters=mbxruntime.parameters.convert(UniqueID), mbxruntime.parameters.convert(ResourceList), mbxruntime.parameters.convert(PivotName),tabledata, TimeStep  EnableBusSupport=off  mask(PreScan Sink Block: VisuMatrixSign){UniqueID=116, ResourceList={'1' 'InformationSign\MatrixSign_GreenArrow.png' '2' 'InformationSign\sign1.jpg' '3' 'InformationSign\sign2.jpg' '4' 'InformationSign\sign3.jpg' '5' 'InformationSign\sign10.png' '7' 'InformationSign\SEARCH_Logo.png' '8' 'InformationSign\sharp_edges.jpg' '9' 'InformationSign\road_surprises.jpg' '10' 'InformationSign\sign5.JPG' '11' 'InformationSign\tacos.jpg' '12' 'InformationSign\dont_even_think.jpg' '13' 'InformationSign\cthulhuwarn.jpg' '14' 'InformationSign\sign7.JPG' '15' 'InformationSign\sign32.jpg' '16' 'InformationSign\NoParking.jpg' '17' 'InformationSign\TheFuture.jpg' '18' 'InformationSign\sign4.jpg' '19' 'InformationSign\sign31.jpg' '20' 'InformationSign\Empty.jpeg' }, PivotName=/child:name=HighwayOverhang_7.InformationPlate_9/trafficSignElement, TimeStep=1/100}
      mask prompts: UniqueID "Parent Unique Identifier (auto-generated)"; ResourceList "Resource List (auto-generated)"; PivotName "Name of pivot (auto-generated)"; TimeStep "Simulink time step"
      mask help:
      | The VisuMatrixSign block provides a way to adapt the texture of the plates connected to an overhang, based on Resource IDs of the texture files.
      |
      | For more information, please click Help.
      mask init:
      | [tabledata] = mbxruntime.parameters.table(UniqueID,ResourceList,PivotName);
      mask Help: eval('openHelp(733)')
      mask Display: image(imread('HighwaySpeedMatrix.png'))
  wires:
  VISUMatrixSign_HighwayOverhang_7/1 -> DemuxVisuMatrixSign/1
  DemuxVisuMatrixSign/1 -> visu_InformationPlate_9/1
  DemuxVisuMatrixSign/2 -> visu_InformationPlate_10/1

== system ACC_Scenario_006_cs/VISUMatrixSign_HighwayOverhang_8/Actuator ==
  VISUMatrixSign_HighwayOverhang_8 : Inport  Tag=inport/VisuMatrixSign  SampleTime=1/100  BusOutputAsStruct=on
  DemuxVisuMatrixSign : Demux  Outputs=2
  visu_InformationPlate_11 : S-Function  FunctionName=sfun_ResourceNameSelector  Parameters=mbxruntime.parameters.convert(UniqueID), mbxruntime.parameters.convert(ResourceList), mbxruntime.parameters.convert(PivotName),tabledata, TimeStep  EnableBusSupport=off  mask(PreScan Sink Block: VisuMatrixSign){UniqueID=117, ResourceList={'1' 'InformationSign\MatrixSign_GreenArrow.png' '2' 'InformationSign\sign1.jpg' '3' 'InformationSign\sign2.jpg' '4' 'InformationSign\sign3.jpg' '5' 'InformationSign\sign10.png' '7' 'InformationSign\SEARCH_Logo.png' '8' 'InformationSign\sharp_edges.jpg' '9' 'InformationSign\road_surprises.jpg' '10' 'InformationSign\sign5.JPG' '11' 'InformationSign\tacos.jpg' '12' 'InformationSign\dont_even_think.jpg' '13' 'InformationSign\cthulhuwarn.jpg' '14' 'InformationSign\sign7.JPG' '15' 'InformationSign\sign32.jpg' '16' 'InformationSign\NoParking.jpg' '17' 'InformationSign\TheFuture.jpg' '18' 'InformationSign\sign4.jpg' '19' 'InformationSign\sign31.jpg' '20' 'InformationSign\Empty.jpeg' }, PivotName=/child:name=HighwayOverhang_8.InformationPlate_11/trafficSignElement, TimeStep=1/100}
      mask prompts: UniqueID "Parent Unique Identifier (auto-generated)"; ResourceList "Resource List (auto-generated)"; PivotName "Name of pivot (auto-generated)"; TimeStep "Simulink time step"
      mask help:
      | The VisuMatrixSign block provides a way to adapt the texture of the plates connected to an overhang, based on Resource IDs of the texture files.
      |
      | For more information, please click Help.
      mask init:
      | [tabledata] = mbxruntime.parameters.table(UniqueID,ResourceList,PivotName);
      mask Help: eval('openHelp(733)')
      mask Display: image(imread('HighwaySpeedMatrix.png'))
  visu_InformationPlate_12 : S-Function  FunctionName=sfun_ResourceNameSelector  Parameters=mbxruntime.parameters.convert(UniqueID), mbxruntime.parameters.convert(ResourceList), mbxruntime.parameters.convert(PivotName),tabledata, TimeStep  EnableBusSupport=off  mask(PreScan Sink Block: VisuMatrixSign){UniqueID=117, ResourceList={'1' 'InformationSign\MatrixSign_GreenArrow.png' '2' 'InformationSign\sign1.jpg' '3' 'InformationSign\sign2.jpg' '4' 'InformationSign\sign3.jpg' '5' 'InformationSign\sign10.png' '7' 'InformationSign\SEARCH_Logo.png' '8' 'InformationSign\sharp_edges.jpg' '9' 'InformationSign\road_surprises.jpg' '10' 'InformationSign\sign5.JPG' '11' 'InformationSign\tacos.jpg' '12' 'InformationSign\dont_even_think.jpg' '13' 'InformationSign\cthulhuwarn.jpg' '14' 'InformationSign\sign7.JPG' '15' 'InformationSign\sign32.jpg' '16' 'InformationSign\NoParking.jpg' '17' 'InformationSign\TheFuture.jpg' '18' 'InformationSign\sign4.jpg' '19' 'InformationSign\sign31.jpg' '20' 'InformationSign\Empty.jpeg' }, PivotName=/child:name=HighwayOverhang_8.InformationPlate_12/trafficSignElement, TimeStep=1/100}
      mask prompts: UniqueID "Parent Unique Identifier (auto-generated)"; ResourceList "Resource List (auto-generated)"; PivotName "Name of pivot (auto-generated)"; TimeStep "Simulink time step"
      mask help:
      | The VisuMatrixSign block provides a way to adapt the texture of the plates connected to an overhang, based on Resource IDs of the texture files.
      |
      | For more information, please click Help.
      mask init:
      | [tabledata] = mbxruntime.parameters.table(UniqueID,ResourceList,PivotName);
      mask Help: eval('openHelp(733)')
      mask Display: image(imread('HighwaySpeedMatrix.png'))
  wires:
  VISUMatrixSign_HighwayOverhang_8/1 -> DemuxVisuMatrixSign/1
  DemuxVisuMatrixSign/1 -> visu_InformationPlate_11/1
  DemuxVisuMatrixSign/2 -> visu_InformationPlate_12/1

== system ACC_Scenario_006_cs/VISUMatrixSign_HighwayOverhang_9/Actuator ==
  VISUMatrixSign_HighwayOverhang_9 : Inport  Tag=inport/VisuMatrixSign  SampleTime=1/100  BusOutputAsStruct=on
  DemuxVisuMatrixSign : Demux  Outputs=2
  visu_InformationPlate_13 : S-Function  FunctionName=sfun_ResourceNameSelector  Parameters=mbxruntime.parameters.convert(UniqueID), mbxruntime.parameters.convert(ResourceList), mbxruntime.parameters.convert(PivotName),tabledata, TimeStep  EnableBusSupport=off  mask(PreScan Sink Block: VisuMatrixSign){UniqueID=118, ResourceList={'1' 'InformationSign\MatrixSign_GreenArrow.png' '2' 'InformationSign\sign1.jpg' '3' 'InformationSign\sign2.jpg' '4' 'InformationSign\sign3.jpg' '5' 'InformationSign\sign10.png' '7' 'InformationSign\SEARCH_Logo.png' '8' 'InformationSign\sharp_edges.jpg' '9' 'InformationSign\road_surprises.jpg' '10' 'InformationSign\sign5.JPG' '11' 'InformationSign\tacos.jpg' '12' 'InformationSign\dont_even_think.jpg' '13' 'InformationSign\cthulhuwarn.jpg' '14' 'InformationSign\sign7.JPG' '15' 'InformationSign\sign32.jpg' '16' 'InformationSign\NoParking.jpg' '17' 'InformationSign\TheFuture.jpg' '18' 'InformationSign\sign4.jpg' '19' 'InformationSign\sign31.jpg' '20' 'InformationSign\Empty.jpeg' }, PivotName=/child:name=HighwayOverhang_9.InformationPlate_13/trafficSignElement, TimeStep=1/100}
      mask prompts: UniqueID "Parent Unique Identifier (auto-generated)"; ResourceList "Resource List (auto-generated)"; PivotName "Name of pivot (auto-generated)"; TimeStep "Simulink time step"
      mask help:
      | The VisuMatrixSign block provides a way to adapt the texture of the plates connected to an overhang, based on Resource IDs of the texture files.
      |
      | For more information, please click Help.
      mask init:
      | [tabledata] = mbxruntime.parameters.table(UniqueID,ResourceList,PivotName);
      mask Help: eval('openHelp(733)')
      mask Display: image(imread('HighwaySpeedMatrix.png'))
  visu_InformationPlate_14 : S-Function  FunctionName=sfun_ResourceNameSelector  Parameters=mbxruntime.parameters.convert(UniqueID), mbxruntime.parameters.convert(ResourceList), mbxruntime.parameters.convert(PivotName),tabledata, TimeStep  EnableBusSupport=off  mask(PreScan Sink Block: VisuMatrixSign){UniqueID=118, ResourceList={'1' 'InformationSign\MatrixSign_GreenArrow.png' '2' 'InformationSign\sign1.jpg' '3' 'InformationSign\sign2.jpg' '4' 'InformationSign\sign3.jpg' '5' 'InformationSign\sign10.png' '7' 'InformationSign\SEARCH_Logo.png' '8' 'InformationSign\sharp_edges.jpg' '9' 'InformationSign\road_surprises.jpg' '10' 'InformationSign\sign5.JPG' '11' 'InformationSign\tacos.jpg' '12' 'InformationSign\dont_even_think.jpg' '13' 'InformationSign\cthulhuwarn.jpg' '14' 'InformationSign\sign7.JPG' '15' 'InformationSign\sign32.jpg' '16' 'InformationSign\NoParking.jpg' '17' 'InformationSign\TheFuture.jpg' '18' 'InformationSign\sign4.jpg' '19' 'InformationSign\sign31.jpg' '20' 'InformationSign\Empty.jpeg' }, PivotName=/child:name=HighwayOverhang_9.InformationPlate_14/trafficSignElement, TimeStep=1/100}
      mask prompts: UniqueID "Parent Unique Identifier (auto-generated)"; ResourceList "Resource List (auto-generated)"; PivotName "Name of pivot (auto-generated)"; TimeStep "Simulink time step"
      mask help:
      | The VisuMatrixSign block provides a way to adapt the texture of the plates connected to an overhang, based on Resource IDs of the texture files.
      |
      | For more information, please click Help.
      mask init:
      | [tabledata] = mbxruntime.parameters.table(UniqueID,ResourceList,PivotName);
      mask Help: eval('openHelp(733)')
      mask Display: image(imread('HighwaySpeedMatrix.png'))
  wires:
  VISUMatrixSign_HighwayOverhang_9/1 -> DemuxVisuMatrixSign/1
  DemuxVisuMatrixSign/1 -> visu_InformationPlate_13/1
  DemuxVisuMatrixSign/2 -> visu_InformationPlate_14/1

== system ACC_Scenario_006_cs/Wheel0_Honda_Pan_European_1/Actuator ==
  Joint : Inport
  Bus Selector : BusSelector  OutputSignals=POSITION,ORIENTATION
  visu_Rotate : Subsystem  mask(RPYActuator){UniqueID=UniqueID, Object3DID=Rotate_ObjectID3D, TimeStep=TimeStep}
      mask prompts: UniqueID "Auto-Assigned: Unique ID"; Object3DID "Auto-Assigned: Child 3D Object ID"; TimeStep "Auto-Assigned: Upload Period [s]"
      mask help: Applies angles update to selected child object
      mask Help:
      | Applies position update to selected child object
      | 
      | - UniqueID (double)   : Unique ID of the parent actor
      | - Object3DID (string) : Name of the child 3D object
      mask Display: port_label('input', 1, ['visu_Rotate_' Object3DID])
  visu_Translate : Subsystem  mask(PositionActuator){UniqueID=UniqueID, Object3DID=Translate_ObjectID3D, TimeStep=TimeStep}
      mask prompts: UniqueID "Auto-Assigned: Unique ID"; Object3DID "Auto-Assigned: Child 3D Object ID"; TimeStep "Auto-Assigned: Upload Period [s]"
      mask help: Applies position update to selected child object
      mask Help:
      | Applies position update to selected child object
      | 
      | - UniqueID (double)   : Unique ID of the parent actor
      | - Object3DID (string) : Name of the child 3D object
      mask Display: port_label('input', 1, ['visu_Translate_' Object3DID])
  wires:
  Bus Selector/2 -> visu_Rotate/1(In1)  "<ORIENTATION>"
  Bus Selector/1 -> visu_Translate/1(In1)  "<POSITION>"
  Joint/1 -> Bus Selector/1
